simulink library "identextras"  (Simulink 7.1)
settings Model: Creator=greg  LastModifiedBy=rsingh

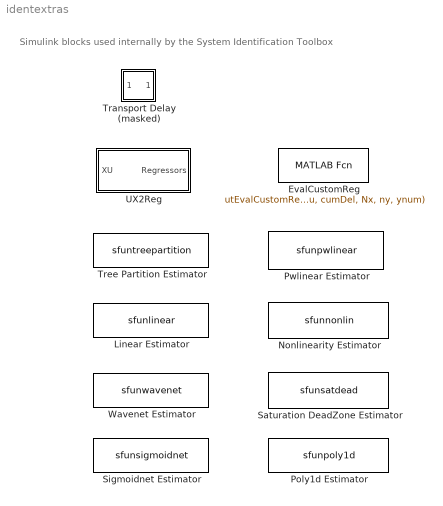
== system identextras ==
  note: Simulink blocks used internally by
      | the System Identification Toolbox
  EvalCustomReg : MATLABFcn  MATLABFcn=utEvalCustomReg(ModelVar, u, cumDel, Nx, ny, ynum)
  Linear Estimator : S-Function  FunctionName=sfunlinear  Parameters=Ts, NumReg, OutputOffset, LinearCoef  SFunctionModules=eval_linear  EnableBusSupport=off  mask(Linear Function){Ts=1, Y0=[], NumReg=1, OutputOffset=0, LinearCoef=0}
      mask prompts: Ts "Sampling time"; Y0 "Initial output values"; NumReg "Number of regressors"; OutputOffset "Model Par: OutputOffset"; LinearCoef "Model Par: LinearCoef"
      mask Display: disp('Linear')
  Nonlinearity Estimator : S-Function  FunctionName=sfunnonlin  Parameters=Ts, NumReg, NonlinObj  EnableBusSupport=off  mask(NEURALNET or CUSTOMNET Estimator){Ts=1, NumReg=1, sys=[], CInd=1, NLType=0}
      mask prompts: Ts "Sampling time"; NumReg "Number of regressors"; sys "Model name"; CInd "Channel Index"; NLType "Input or Output NL (for IDNLHW)"
      mask help: Simulate the output of a NEURALNET or CUSTOMNET nonlinearity estimator.
      mask init:
      | sysname = 'Generic Nonlinearity';
      | if isa(sys,'idnlarx')
      |     NonlinObj = sys.Nonlinearity;
      | elseif isa(sys,'idnlhw')
      |     if strcmpi(NLType,'Input')
      |         NonlinObj = sys.InputNonlinearity;
      |     else
      |         NonlinObj = sys.OutputNonlinearity;
      |     end
      | else
      |     NonlinObj = [];
      | end
      | 
      | if ~isempty(NonlinObj)
      |     NonlinObj = NonlinObj(CInd);
      |     if isa(NonlinObj,'neuralnet')
      |         sysname = 'Neural Network';
      |     elseif isa(NonlinObj,'customnet')
      |         sysname = 'Custom Network';
      |     end
      | end
      mask Help:
      | Code generation using RTW is not possible when using this block.
      | If nonlinearity is NEURALNET, Neural Network Toolbox is required in order to perform simulation.
      mask Display: disp(sysname)
  Poly1d Estimator : S-Function  FunctionName=sfunpoly1d  Parameters=Ts, Degree, Coefficients  SFunctionModules=eval_poly1d  EnableBusSupport=off  mask(Poly1d Estimator){Ts=1, Degree=0, Coefficients=[]}
      mask prompts: Ts "Sampling time"
      mask help: Simulate the response of a one-dimensional polynomial estimator used for Hammerstein-Wiener models.
      mask Display: disp('1-D Polynomial')
  Pwlinear Estimator : S-Function  FunctionName=sfunpwlinear  Parameters=Ts, NumReg, NumUnits, LinearCoef, OutputOffset, OutputCoef, Translation  SFunctionModules=eval_pwlinear  EnableBusSupport=off  mask{Ts=1, NumReg=1, NumUnits=0, LinearCoef=0, OutputOffset=0, OutputCoef=0, Translation=0}
      mask prompts: Ts "Sampling time"; NumReg "Number of regressors (should be 1)"; NumUnits "Model Par: NumUnits"; LinearCoef "Model Par: LinearCoef"; OutputOffset "Model Par: OutputOffset"; OutputCoef "Model Par: OutputCoef"; Translation "Model Par: Translation"
      mask Display: disp('Piecewise Linear')
  Saturation DeadZone Estimator : S-Function  FunctionName=sfunsatdead  Parameters=Ts, Interval, Center, Scale, IsSaturation  SFunctionModules=eval_satdead  EnableBusSupport=off  mask(Saturation or DeadZone Estimator){Ts=1, Interval=[], Center=0, Scale=0, IsSaturation=1}
      mask prompts: Ts "Sampling time"; Interval "Interval (linear or dead)"; IsSaturation "Does this block represent saturation?"
      mask init:
      | if IsSaturation==1
      |     sysname = 'Saturation';
      | else
      |     sysname = 'DeadZone';
      | end
      mask Display: disp(sysname)
  Sigmoidnet Estimator : S-Function  FunctionName=sfunsigmoidnet  Parameters=Ts, NumReg, NumUnits, RegressorMean, NonLinearSubspace, LinearSubspace, LinearCoef, Dilation, Translation, OutputCoef, OutputOffset  SFunctionModules=eval_sigmoidnet  EnableBusSupport=off  mask{Ts=1, NumReg=1, NumUnits=0, RegressorMean=0, NonLinearSubspace=0, LinearSubspace=0, LinearCoef=0, Dilation=0, Translation=0, OutputCoef=0, OutputOffset=0}
      mask prompts: Ts "Sampling time"; NumReg "Number of regressors"; NumUnits "Model Par: NumUnits"; RegressorMean "Model Par: RegressorMean"; NonLinearSubspace "Model Par: NonLinearSubspace"; LinearSubspace "Model Par: LinearSubspace"; LinearCoef "Model Par: LinearCoef"; Dilation "Model Par: Dilation"; Translation "Model Par: Translation"; OutputCoef "Model Par: OutputCoef"; OutputOffset "Model Par: OutputOffset"
      mask Display: disp('Sigmoid Network')
  Transport Delay (masked) : Subsystem  mask(Transport Delay (masked)){Td=1, u0=0, bufsize=1024}
      mask prompts: Td "Delay Time"; u0 "Initial Input"; bufsize "Initial Buffer Size"
      mask help: Transport Delay, with direct feedthrough when Delay Time is equal to zero.
      mask init:
      | df = get_param(bdroot,'dirty');
      | iddfthru(gcb, Td, u0, bufsize);
      | set_param(bdroot,'dirty',df)
      mask Help: See Transport Delay for more information.
      mask Display: block_icon('Transport Delay')
  Tree Partition Estimator : S-Function  FunctionName=sfuntreepartition  Parameters=Ts, NumReg, NumUnits, RegressorMean, OutputOffset, LinearCoef, SampleLength, NoiseVariance, TreeLevelPntr, AncestorDescendantPntr, LocalizingVectors, LocalCovMatrix, LocalParVector, Threshold  SFunctionModules=eval_treepartition  EnableBusSupport=off  mask(Tree Partition Function){Ts=1, NumReg=1, NumUnits=0, RegressorMean=0, OutputOffset=0, LinearCoef=0, SampleLength=0, NoiseVariance=0, TreeLevelPntr=0, AncestorDescendantPntr=0, LocalizingVectors=0, LocalCovMatrix=0, LocalParVector=0, Threshold=1}
      mask prompts: Ts "Sampling time"; NumReg "Number of regressors"; NumUnits "Model Par: NumUnits"; RegressorMean "Model Par: RegressorMean"; OutputOffset "Model Par: OutputOffset"; LinearCoef "Model Par: LinearCoef"; SampleLength "Model Par: SampleLength"; NoiseVariance "Model Par: NoiseVariance"; TreeLevelPntr "Model Par: TreeLevelPntr"; AncestorDescendantPntr "Model Par: AncestorDescendantPntr"; LocalizingVectors "Model Par: LocalizingVectors"; LocalCovMatrix "Model Par: LocalCovMatrix"; LocalParVector "Model Par: LocalParVector"; Threshold "Model Par: Threshold"
      mask Display: disp('Tree Partition')
  UX2Reg : Subsystem  mask(Generate Regressors){ny=1, Nx=0, ynum=1, cumDel=0, ModelVar=[], K=0}
      mask prompts: ny "Total number of outputs"; Nx "Number of states"; ynum "This output index"; cumDel "Cumulative Delay for this output"; ModelVar "Model variable ([] if no custom reg)"; K "Regressor selector (matrix gain)"
      mask help: Generate regressors from input and state variables.
      mask Help: Utility used by Nonlinear ARX model block.
      mask Display:
      | port_label('input',1,'XU')
      | port_label('output',1,'Regressors')
  Wavenet Estimator : S-Function  FunctionName=sfunwavenet  Parameters=Ts, NumReg, NumUnits, RegressorMean, NonLinearSubspace, LinearSubspace, OutputOffset, LinearCoef, ScalingCoef, WaveletCoef, ScalingDilation, WaveletDilation, ScalingTranslation, WaveletTranslation  SFunctionModules=eval_wavenet  EnableBusSupport=off  mask{Ts=1, NumReg=1, NumUnits=0, RegressorMean=0, NonLinearSubspace=0, LinearSubspace=0, OutputOffset=0, LinearCoef=0, ScalingCoef=0, WaveletCoef=0, ScalingDilation=0, WaveletDilation=0, ScalingTranslation=0, WaveletTranslation=0}
      mask prompts: Ts "Sampling time"; NumReg "Number of regressors"; NumUnits "Model Par: NumUnits"; RegressorMean "Model Par: RegressorMean"; NonLinearSubspace "Model Par: NonLinearSubspace"; LinearSubspace "Model Par: LinearSubspace"; OutputOffset "Model Par: OutputOffset"; LinearCoef "Model Par: LinearCoef"; ScalingCoef "Model Par: ScalingCoef"; WaveletCoef "Model Par: WaveletCoef"; ScalingDilation "Model Par: ScalingDilation"; WaveletDilation "Model Par: WaveletDilation"; ScalingTranslation "Model Par: ScalingTranslation"; WaveletTranslation "Model Par: WaveletTranslation"
      mask Display: disp('Wavelet Network')

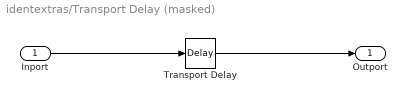
== system identextras/Transport Delay (masked) ==
  Inport : Inport  OutDataType=sfix(16)  OutScaling=2^0
  Transport Delay : TransportDelay
  Outport : Outport  OutDataType=sfix(16)  OutScaling=2^0
  wires:
  Inport/1 -> Transport Delay/1
  Transport Delay/1 -> Outport/1

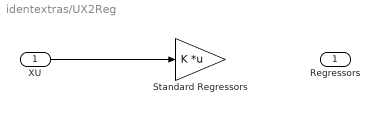
== system identextras/UX2Reg ==
  XU : Inport  OutDataType=sfix(16)  OutScaling=2^0
  Standard Regressors : Gain  Gain=K  Multiplication=Matrix(K*u)  ParameterDataType=sfix(16)  ParameterScaling=2^0  OutDataType=sfix(16)  OutScaling=2^0
  Regressors : Outport  OutDataType=sfix(16)  OutScaling=2^0
  wires:
  XU/1 -> Standard Regressors/1
